simulink model "pid_model"  (R2016b)
settings: Solver=FixedStepAuto  StartTime=0.0  StopTime=10.0  FixedStep=0.1  RelTol=1e-3
settings Model: Creator=vanou  LastModifiedBy=vanou

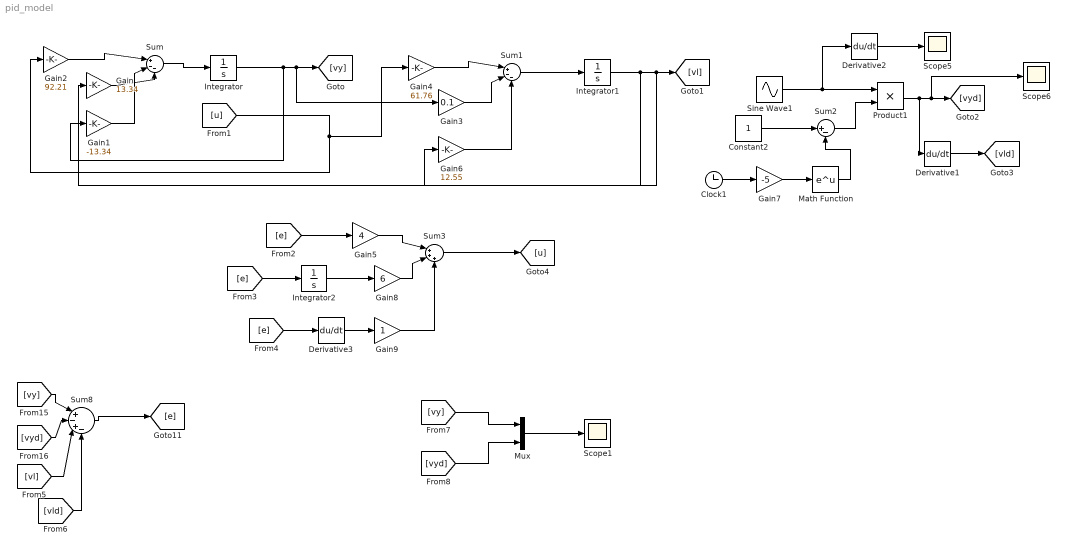
== system pid_model ==
  Clock1 : Clock
  Constant2 : Constant
  Derivative1 : Derivative
  Derivative2 : Derivative
  Derivative3 : Derivative
  Gain : Gain  Gain=13.34
  Gain1 : Gain  Gain=-13.34
  Gain2 : Gain  Gain=92.21
  Gain3 : Gain  Gain=0.1
  Gain4 : Gain  Gain=61.76
  Gain5 : Gain  Gain=4
  Gain6 : Gain  Gain=12.55
  Gain7 : Gain  Gain=-5
  Gain8 : Gain  Gain=6
  Gain9 : Gain
  Integrator : Integrator
  Integrator1 : Integrator
  Integrator2 : Integrator
  Math Function : Math  SaturateOnIntegerOverflow=on
  Mux : Mux  Inputs=2
  Product1 : Product
  Scope1 : Scope
  Scope5 : Scope
  Scope6 : Scope
  Sine Wave1 : Sin  SampleTime=0
  Sum : Sum  Inputs=|+--
  Sum1 : Sum  Inputs=|+--
  Sum2 : Sum  Inputs=|+-
  Sum3 : Sum  Inputs=|+++
  Sum8 : Sum  Inputs=|+-+-
  wires:
  Sum/1 -> Integrator/1
  Gain2/1 -> Sum/1
  Gain1/1 -> Sum/2
  Gain/1 -> Sum/3
  Sum1/1 -> Integrator1/1
  Gain4/1 -> Sum1/1
  Gain3/1 -> Sum1/2
  Integrator/1 -> Gain1/1, Gain3/1, [vy]
  [u] -> Gain2/1, Gain4/1
  Gain6/1 -> Sum1/3
  Integrator1/1 -> Gain6/1, Gain/1, [vl]
  Clock1/1 -> Gain7/1
  Gain7/1 -> Math Function/1
  Sine Wave1/1 -> Derivative2/1, Product1/1
  Math Function/1 -> Sum2/2
  Constant2/1 -> Sum2/1
  Sum2/1 -> Product1/2
  Product1/1 -> Derivative1/1, Scope6/1, [vyd]
  Derivative1/1 -> [vld]
  [vy] -> Sum8/1
  [vyd] -> Sum8/2
  Sum8/1 -> [e]
  Derivative2/1 -> Scope5/1
  [e] -> Gain5/1
  [e] -> Integrator2/1
  Gain5/1 -> Sum3/1
  [e] -> Derivative3/1
  Integrator2/1 -> Gain8/1
  Gain8/1 -> Sum3/2
  Derivative3/1 -> Gain9/1
  Gain9/1 -> Sum3/3
  Sum3/1 -> [u]
  [vl] -> Sum8/3
  [vld] -> Sum8/4
  [vy] -> Mux/1
  [vyd] -> Mux/2
  Mux/1 -> Scope1/1
